simulink model "CalculateAvgColors"  (R2016a)
settings: Solver=VariableStepAuto  StartTime=0.0  StopTime=0  RelTol=1e-3
undefined symbols (not defined in the file or in its folder): Rec, SDTV
libraries: visionconversions x3, visionsources x1
settings Model: Creator=Lakmini  LastModifiedBy=Lakmini

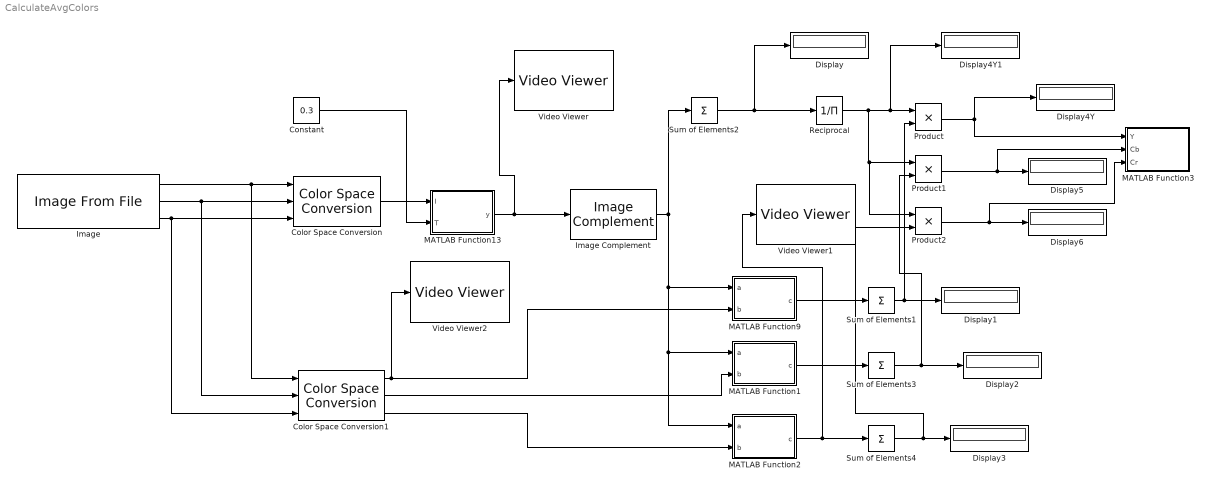
== system CalculateAvgColors ==
  Color Space Conversion : visionconversions/Color Space  Conversion  conversion=Obsolete  conversionActive=R'G'B' to intensity  wp_str=D65  rec=Rec. 601 (SDTV)  sys=1125/60/2:1  imagePorts=Separate color signals
  Color Space Conversion1 : visionconversions/Color Space  Conversion  conversion=Obsolete  conversionActive=R'G'B' to Y'CbCr  wp_str=D65  rec=Rec. 601 (SDTV)  sys=1125/60/2:1  imagePorts=Separate color signals
  Constant : Constant  Value=0.3  OutDataTypeStr=double  SampleTime=1
  Display{,1..3,5..6} (6 alike) : Display
  Display4Y : Display
  Display4Y1 : Display
  "Image " : visionsources/Image From File  Tag=vipblks_nd  FileName=E:\Acadamic\Semester7\FYP\bluelight\New folder\a_leaf\Blue_Leaf15.jpg  imagePorts=Separate color signals  Ts=1  ImageDataType=Inherit from input image  Signed=on  WordLength=16  sdImageDataType=uint(8)  FractionLengthMode=User-defined  FractionLength=15  OutPortLabels=R|G|B
  Image Complement : visionconversions/Image Complement
  MATLAB Function1 : MATLAB Function  TreatAsAtomicUnit=on
  MATLAB Function13 : MATLAB Function  TreatAsAtomicUnit=on
  MATLAB Function2 : MATLAB Function  TreatAsAtomicUnit=on
  MATLAB Function3 : MATLAB Function  TreatAsAtomicUnit=on
  MATLAB Function9 : MATLAB Function  TreatAsAtomicUnit=on
  Product : Product  OutDataTypeStr=double
  Product1 : Product  OutDataTypeStr=double
  Product2 : Product  OutDataTypeStr=double
  Reciprocal : Product  Inputs=/  OutDataTypeStr=double  SaturateOnIntegerOverflow=on  RndMeth=Zero
  Sum of Elements1 : Sum  Inputs=+  AccumDataTypeStr=double  OutDataTypeStr=double
  Sum of Elements2 : Sum  Inputs=+  AccumDataTypeStr=double  OutDataTypeStr=double  RndMeth=Nearest
  Sum of Elements3 : Sum  Inputs=+  AccumDataTypeStr=double  OutDataTypeStr=double
  Sum of Elements4 : Sum  Inputs=+  AccumDataTypeStr=double  OutDataTypeStr=double
  Video Viewer : VideoViewer  FigPos=[1 726 1362 626]
  Video Viewer1 : VideoViewer  FigPos=[613 734 667 611]
  Video Viewer2 : VideoViewer  FigPos=[613 734 667 611]
  wires:
  Color Space Conversion/1 -> MATLAB Function13/1(I)
  Constant/1 -> MATLAB Function13/2(T)
  MATLAB Function13/1(y) -> Video Viewer/1, Image Complement/1
  Sum of Elements2/1 -> Reciprocal/1, Display/1
  Image Complement/1 -> MATLAB Function2/1(a), MATLAB Function1/1(a), MATLAB Function9/1(a), Sum of Elements2/1
  "Image "/1 -> Color Space Conversion1/1, Color Space Conversion/1
  "Image "/3 -> Color Space Conversion1/3, Color Space Conversion/3
  "Image "/2 -> Color Space Conversion1/2, Color Space Conversion/2
  MATLAB Function9/1(c) -> Sum of Elements1/1
  MATLAB Function1/1(c) -> Sum of Elements3/1
  MATLAB Function2/1(c) -> Video Viewer1/1, Sum of Elements4/1
  Sum of Elements3/1 -> Product1/2, Display2/1
  Sum of Elements1/1 -> Product/2, Display1/1
  Sum of Elements4/1 -> Product2/2, Display3/1
  Reciprocal/1 -> Product2/1, Product1/1, Display4Y1/1, Product/1
  Product/1 -> MATLAB Function3/1(Y), Display4Y/1
  Product1/1 -> MATLAB Function3/2(Cb), Display5/1
  Product2/1 -> MATLAB Function3/3(Cr), Display6/1
  Color Space Conversion1/1 -> Video Viewer2/1, MATLAB Function9/2(b)
  Color Space Conversion1/2 -> MATLAB Function1/2(b)
  Color Space Conversion1/3 -> MATLAB Function2/2(b)

== matlab function CalculateAvgColors/MATLAB Function1 ==
  data: a input; b input; c output
function c = fcn(a,b)
%#codegen
c=uint8(a).*b;
return

== matlab function CalculateAvgColors/MATLAB Function2 ==
  data: a input; b input; c output
function c = fcn(a,b)
%#codegen
c=uint8(a).*uint8(b);
return

== matlab function CalculateAvgColors/MATLAB Function3 ==
  data: Y input; Cb input; Cr input
function fcn(Y,Cb,Cr)
coder.extrinsic('xlsread');
coder.extrinsic('size');
coder.extrinsic('num2str');
coder.extrinsic('strcat');
coder.extrinsic('xlswrite');
a = xlsread('E:\testdata_blueLight.xlsx');
% new data to write in file
t = {Y,Cb,Cr};
nRows=0;
% last row with data in the file
nRows = (size(a,1));


% plus 1 to write in the next line (if you have an header it should be + 2)
nRows = nRows +2;

% convert number to string
b = num2str(nRows)

% if you want to add data to the collum A you make concat strings
c = strcat('A', b)

% right to file the data t on the sheet Folha1 begining in the row c (e.g. A20)
xlswrite('E:\testdata_blueLight.xlsx', t,'sheet1',c);

 

end

== matlab function CalculateAvgColors/MATLAB Function13 ==
  data: I input; y output; T input
function y = fcn(I,T)
%#codegen
BW = imbinarize(I,double(T));
y = BW;
coder.extrinsic('display');
display(y);

== matlab function CalculateAvgColors/MATLAB Function9 ==
  data: a input; b input; c output
function c = fcn(a,b)
%#codegen
c=uint8(a).*b;
disp(c)
return
